simulink model "secante"  (R2017a)
settings: Solver=VariableStepAuto  StartTime=0.0  StopTime=inf  RelTol=1e-3
values from neighbouring files (symbols this model uses):
  tol = 1e-3    (= 0.001)    [metodoSecante.m]
  x0 = -3    [metodoSecante.m]
  x1 = 5    [metodoSecante.m]
libraries: simulink x1
settings Model: Creator=Enrico Donato  LastModifiedBy=Enrico Donato

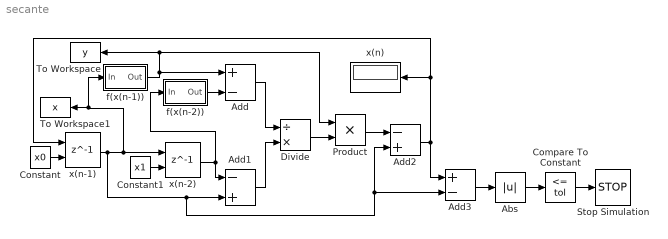
== system secante ==
  Abs : Abs
  Add : Sum  Inputs=+-
  Add1 : Sum  Inputs=-+
  Add2 : Sum  Inputs=-+
  Add3 : Sum  Inputs=+-
  Compare To Constant : simulink/Logic and Bit Operations/Compare To Constant  relop=<=  const=tol  OutDataTypeStr=boolean
  Constant : Constant  Value=x0
  Constant1 : Constant  Value=x1
  Divide : Product  Inputs=/*
  Product : Product
  Stop Simulation : Stop
  To Workspace : ToWorkspace  VariableName=y  SampleTime=-1
      settings: Save2DSignal=2-D array (concatenate along first dimension)
  To Workspace1 : ToWorkspace  VariableName=x  SampleTime=-1
  f(x(n-1)) : Subsystem
  f(x(n-2)) : Subsystem
  x(n) : Display
  x(n-1) : Delay  DelayLength=1  InitialConditionSource=Input port  InitialCondition=0  SampleTime=1
      settings: InputPortMap=u0,p4
  x(n-2) : Delay  DelayLength=1  InitialConditionSource=Input port  InitialCondition=0  SampleTime=1
      settings: InputPortMap=u0,p4
  wires:
  Constant1/1 -> x(n-2)/2
  Constant/1 -> x(n-1)/2
  x(n-2)/1 -> Add1/1, f(x(n-2))/1(In)
  f(x(n-2))/1(Out) -> Add/2
  Add1/1 -> Divide/2
  Add/1 -> Divide/1
  Divide/1 -> Product/2
  Product/1 -> Add2/1
  x(n-1)/1 -> Add3/2, Add2/2, Add1/2, x(n-2)/1, To Workspace1/1, f(x(n-1))/1(In)
  Add2/1 -> Add3/1, x(n-1)/1, x(n)/1
  Compare To Constant/1 -> Stop Simulation/1
  Add3/1 -> Abs/1
  Abs/1 -> Compare To Constant/1
  f(x(n-1))/1(Out) -> Product/1, To Workspace/1, Add/1

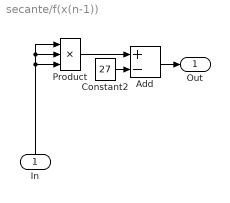
== system secante/f(x(n-1)) ==
  In : Inport
  Add : Sum  Inputs=+-
  Constant2 : Constant  Value=27
  Product : Product  Inputs=3
  Out : Outport
  wires:
  Add/1 -> Out/1
  In/1 -> Product/3, Product/2, Product/1
  Product/1 -> Add/1
  Constant2/1 -> Add/2

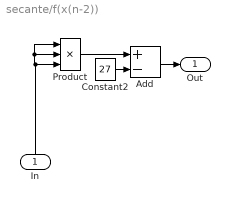
== system secante/f(x(n-2)) ==
  In : Inport
  Add : Sum  Inputs=+-
  Constant2 : Constant  Value=27
  Product : Product  Inputs=3
  Out : Outport
  wires:
  Add/1 -> Out/1
  In/1 -> Product/2, Product/1, Product/3
  Product/1 -> Add/1
  Constant2/1 -> Add/2
